simulink model "Simulation_simulink"  (R2024a)
settings: Solver=VariableStepAuto  StartTime=0.0  StopTime=reference.tsim  RelTol=1e-3
values from neighbouring files (symbols this model uses):
  Alat = Inlat_inv*Alat_    [create_sf_lti.m]
  Alon = Inlon_inv*Alon_    [create_sf_lti.m]
  Blat = Inlat_inv*Blat_    [create_sf_lti.m]
  Blon = Inlon_inv*Blon_    [create_sf_lti.m]
  Kd_psi = 10    [Mh03_h1000.m]    (also in demo.m)
  Kd_roll = -10    [Mh03_h1000.m]    (also in demo.m)
  Ki_pitch = -0.1    [Mh03_h1000.m]    (also in demo.m)
  Ki_psi = 0.1    [Mh03_h1000.m]    (also in demo.m)
  Kp = -4.7989    [Mh03_h1000.m]    (also in controller_1.m = evalin("base", "Kp"); demo.m)
  Kp_pitch = -10    [Mh03_h1000.m]    (also in demo.m = -1)
  Kp_psi = 10    [Mh03_h1000.m]    (also in demo.m)
  Kp_roll = -1    [Mh03_h1000.m]    (also in demo.m)
  Kq = -100000    [Mh03_h1000.m]    (also in controller_1.m = evalin("base", "Kq"); demo.m = 100)
  Kr = 6.9343    [Mh03_h1000.m]    (also in controller_1.m = evalin("base", "Kr"); demo.m)
  Ksp = 0.1    [Mh03_h1000.m]    (also in demo.m)
  Ksq = 0.1    [Mh03_h1000.m]    (also in demo.m)
  Ksr = 0.1    [Mh03_h1000.m]    (also in demo.m)
  reference = evalin('base', 'reference')    [GravityFM.m]    (also in Mh03_h1000.m = create_sf_reference(); demo.m = create_sf_reference())
  tau_p = 0.5    [Mh03_h1000.m]    (also in demo.m)
  tau_q = 0.5    [Mh03_h1000.m]    (also in demo.m)
  tau_r = 0.5    [Mh03_h1000.m]    (also in demo.m)
undefined symbols (not defined in the file or in its folder): Earth, Kiq, Kpp, Kpq, Kpr, KSp, KSr, WGS84
libraries: slpidlib x2, aerolibtransform2 x1
settings Model: Creator=jelho  LastModifiedBy=ludhor
settings DataIOCC: ExternalInput=getinputstruct(report2)  InitialState=getstatestruct(report2)
settings RTWCC: GPUComputeCapability=3.5

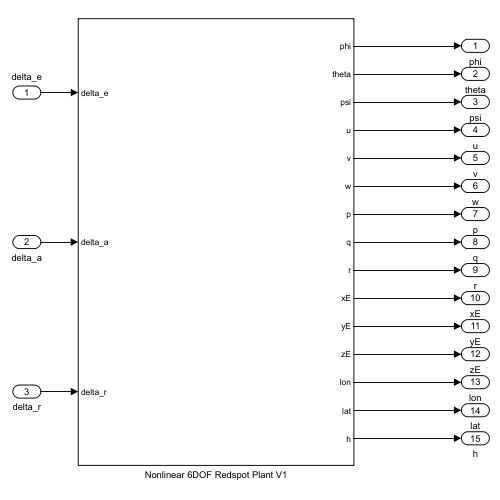
[thumbnail: Simulink's stored preview of the top-level diagram]
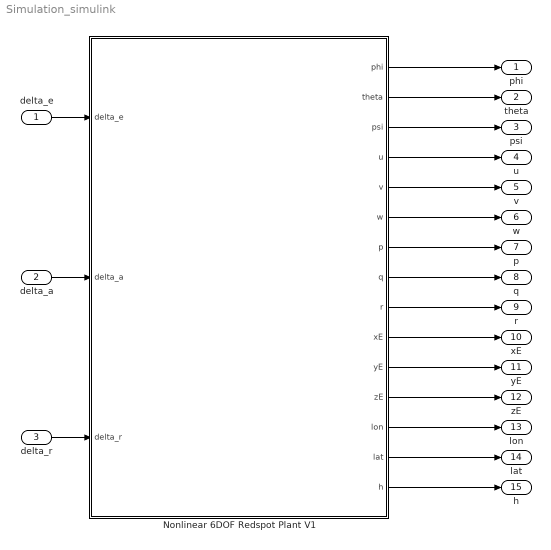
== system Simulation_simulink ==
  delta_e : Inport
  delta_a : Inport  Port=2
  delta_r : Inport  Port=3
  Nonlinear 6DOF Redspot Plant V1 : Subsystem
  phi : Outport
  theta : Outport  Port=2
  psi : Outport  Port=3
  u : Outport  Port=4
  v : Outport  Port=5
  w : Outport  Port=6
  p : Outport  Port=7
  q : Outport  Port=8
  r : Outport  Port=9
  xE : Outport  Port=10
  yE : Outport  Port=11
  zE : Outport  Port=12
  lon : Outport  Port=13
  lat : Outport  Port=14
  h : Outport  Port=15
  wires:
  delta_e/1 -> Nonlinear 6DOF Redspot Plant V1/1(delta_e)
  delta_a/1 -> Nonlinear 6DOF Redspot Plant V1/2(delta_a)
  delta_r/1 -> Nonlinear 6DOF Redspot Plant V1/3(delta_r)
  Nonlinear 6DOF Redspot Plant V1/6(w) -> w/1
  Nonlinear 6DOF Redspot Plant V1/1(phi) -> phi/1
  Nonlinear 6DOF Redspot Plant V1/4(u) -> u/1
  Nonlinear 6DOF Redspot Plant V1/2(theta) -> theta/1
  Nonlinear 6DOF Redspot Plant V1/3(psi) -> psi/1
  Nonlinear 6DOF Redspot Plant V1/5(v) -> v/1
  Nonlinear 6DOF Redspot Plant V1/7(p) -> p/1
  Nonlinear 6DOF Redspot Plant V1/8(q) -> q/1
  Nonlinear 6DOF Redspot Plant V1/9(r) -> r/1
  Nonlinear 6DOF Redspot Plant V1/10(xE) -> xE/1
  Nonlinear 6DOF Redspot Plant V1/11(yE) -> yE/1
  Nonlinear 6DOF Redspot Plant V1/12(zE) -> zE/1
  Nonlinear 6DOF Redspot Plant V1/13(lon) -> lon/1
  Nonlinear 6DOF Redspot Plant V1/14(lat) -> lat/1
  Nonlinear 6DOF Redspot Plant V1/15(h) -> h/1

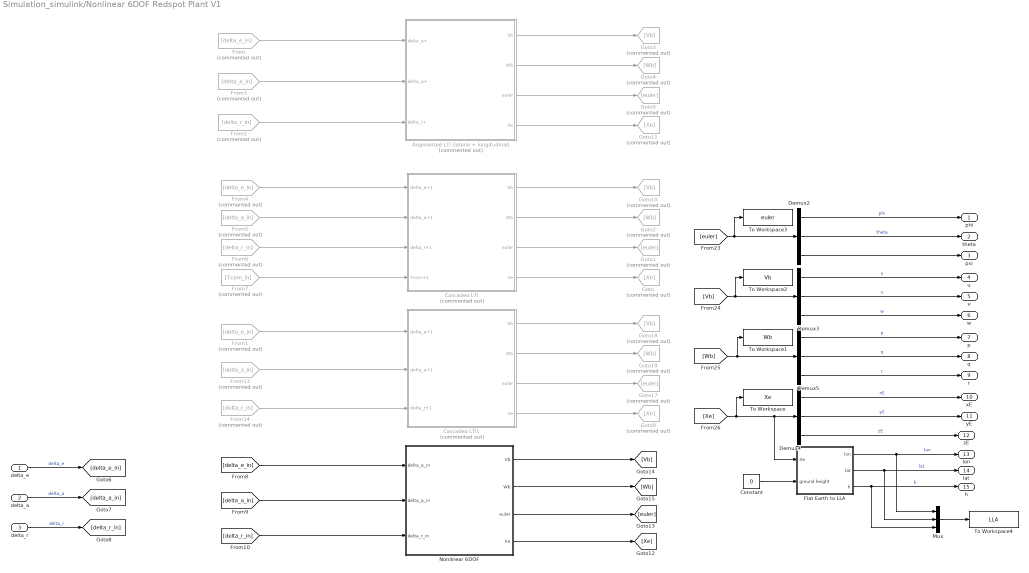
== system Simulation_simulink/Nonlinear 6DOF Redspot Plant V1 ==
  delta_e : Inport
  delta_a : Inport  Port=2
  delta_r : Inport  Port=3
  Augmented LTI (lateral + longitudinal) : Subsystem  Commented=on
  Cascaded LTI : Subsystem  Commented=on
  Cascaded LTI1 : Subsystem  Commented=on
  Constant : Constant  Value=0
  Demux{2..5} (4 alike) : Demux  Outputs=3
  Flat Earth to LLA : Subsystem
  From : From  Commented=on  GotoTag=delta_e_in
  From1 : From  Commented=on  GotoTag=delta_e_in
  From13 : From  Commented=on  GotoTag=delta_a_in
  From14 : From  Commented=on  GotoTag=delta_r_in
  From2 : From  Commented=on  GotoTag=delta_r_in
  From3 : From  Commented=on  GotoTag=delta_a_in
  From4 : From  Commented=on  GotoTag=delta_e_in
  From5 : From  Commented=on  GotoTag=delta_a_in
  From6 : From  Commented=on  GotoTag=delta_r_in
  From7 : From  Commented=on  GotoTag=Tcom_in
  Goto : Goto  Commented=on  GotoTag=Xe
  Goto1 : Goto  Commented=on  GotoTag=euler
  Goto10 : Goto  Commented=on  GotoTag=Vb
  Goto11 : Goto  Commented=on  GotoTag=Xe
  Goto17 : Goto  Commented=on  GotoTag=euler
  Goto18 : Goto  Commented=on  GotoTag=Vb
  Goto19 : Goto  Commented=on  GotoTag=Wb
  Goto2 : Goto  Commented=on  GotoTag=Wb
  Goto3 : Goto  Commented=on  GotoTag=Vb
  Goto4 : Goto  Commented=on  GotoTag=Wb
  Goto5 : Goto  Commented=on  GotoTag=euler
  Goto9 : Goto  Commented=on  GotoTag=Xe
  Mux : Mux  Inputs=3
  Nonlinear 6DOF : Subsystem
  To Workspace : ToWorkspace  VariableName=Xe  SaveFormat=Timeseries  SampleTime=-1
  To Workspace1 : ToWorkspace  VariableName=Wb  SaveFormat=Timeseries  SampleTime=-1
  To Workspace2 : ToWorkspace  VariableName=Vb  SaveFormat=Timeseries  SampleTime=-1
  To Workspace3 : ToWorkspace  VariableName=euler  SaveFormat=Timeseries  SampleTime=-1
  To Workspace4 : ToWorkspace  VariableName=LLA  SaveFormat=Timeseries  SampleTime=-1
  phi : Outport
  theta : Outport  Port=2
  psi : Outport  Port=3
  u : Outport  Port=4
  v : Outport  Port=5
  w : Outport  Port=6
  p : Outport  Port=7
  q : Outport  Port=8
  r : Outport  Port=9
  xE : Outport  Port=10
  yE : Outport  Port=11
  zE : Outport  Port=12
  lon : Outport  Port=13
  lat : Outport  Port=14
  h : Outport  Port=15
  wires:
  delta_a/1 -> [delta_a_in]  "delta_a"
  delta_e/1 -> [delta_e_in]  "delta_e"
  [Vb] -> To Workspace2/1, Demux3/1
  [euler] -> To Workspace3/1, Demux2/1
  delta_r/1 -> [delta_r_in]  "delta_r"
  Demux2/1 -> phi/1  "phi"
  Demux2/2 -> theta/1  "theta"
  Demux2/3 -> psi/1
  Demux3/3 -> w/1  "w"
  Demux3/1 -> u/1  "u"
  Demux3/2 -> v/1  "v"
  Demux5/2 -> q/1  "q"
  [Wb] -> To Workspace1/1, Demux5/1
  Demux5/1 -> p/1  "p"
  Demux5/3 -> r/1  "r"
  [Xe] -> To Workspace/1, Flat Earth to LLA/1(Xe), Demux4/1
  Demux4/2 -> yE/1  "yE"
  Demux4/3 -> zE/1  "zE"
  Demux4/1 -> xE/1  "xE"
  [delta_e_in] -> Nonlinear 6DOF/1(delta_e_in)
  [delta_a_in] -> Nonlinear 6DOF/2(delta_a_in)
  [delta_r_in] -> Nonlinear 6DOF/3(delta_r_in)
  Nonlinear 6DOF/1(Vb) -> [Vb]
  Nonlinear 6DOF/2(Wb) -> [Wb]
  Nonlinear 6DOF/3(euler) -> [euler]
  Nonlinear 6DOF/4(Xe) -> [Xe]
  From4/1 -> Cascaded LTI/1(delta_e+1)
  From5/1 -> Cascaded LTI/2(delta_a+1)
  From6/1 -> Cascaded LTI/3(delta_r+1)
  From7/1 -> Cascaded LTI/4(Tcom+1)
  Cascaded LTI/1(Vb) -> Goto10/1
  Cascaded LTI/2(Wb) -> Goto2/1
  Cascaded LTI/3(euler) -> Goto1/1
  Cascaded LTI/4(Xe) -> Goto/1
  From/1 -> Augmented LTI (lateral + longitudinal)/1(delta_e+)
  From2/1 -> Augmented LTI (lateral + longitudinal)/3(delta_r+)
  From3/1 -> Augmented LTI (lateral + longitudinal)/2(delta_a+)
  Augmented LTI (lateral + longitudinal)/1(Vb) -> Goto3/1
  Augmented LTI (lateral + longitudinal)/2(Wb) -> Goto4/1
  Augmented LTI (lateral + longitudinal)/3(euler) -> Goto5/1
  Augmented LTI (lateral + longitudinal)/4(Xe) -> Goto11/1
  Flat Earth to LLA/1(lon) -> Mux/1, lon/1  "lon"
  Flat Earth to LLA/2(lat) -> Mux/2, lat/1  "lat"
  Flat Earth to LLA/3(h) -> Mux/3, h/1  "h"
  Constant/1 -> Flat Earth to LLA/2(ground height)
  Mux/1 -> To Workspace4/1
  From1/1 -> Cascaded LTI1/1(delta_e+1)
  Cascaded LTI1/4(Xe) -> Goto9/1
  Cascaded LTI1/1(Vb) -> Goto18/1
  From14/1 -> Cascaded LTI1/3(delta_r+1)
  From13/1 -> Cascaded LTI1/2(delta_a+1)
  Cascaded LTI1/3(euler) -> Goto17/1
  Cascaded LTI1/2(Wb) -> Goto19/1

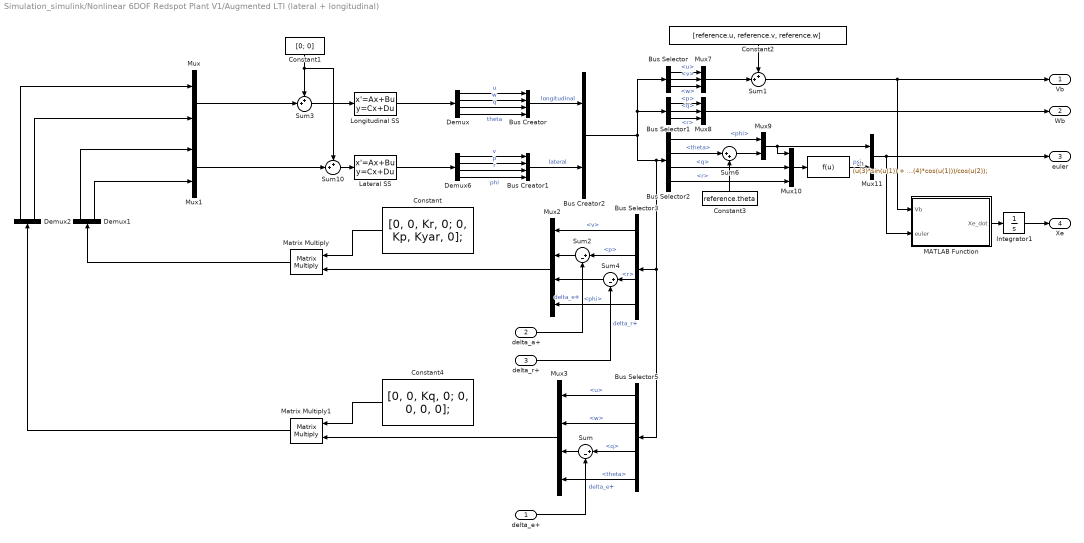
== system Simulation_simulink/Nonlinear 6DOF Redspot Plant V1/Augmented LTI (lateral + longitudinal) ==
  delta_e+ : Inport
  delta_a+ : Inport  Port=2
  delta_r+ : Inport  Port=3
  Bus Creator : BusCreator  Inputs=4
  Bus Creator1 : BusCreator  Inputs=4
  Bus Creator2 : BusCreator  Inputs=2
  Bus Selector : BusSelector  OutputSignals=longitudinal.u,lateral.v,longitudinal.w
  Bus Selector1 : BusSelector  OutputSignals=lateral.p,longitudinal.q,lateral.r
  Bus Selector2 : BusSelector  OutputSignals=lateral.phi,longitudinal.theta,longitudinal.q,lateral.r
  Bus Selector3 : BusSelector  OutputSignals=lateral.v,lateral.p,lateral.r,lateral.phi
  Bus Selector5 : BusSelector  OutputSignals=longitudinal.u,longitudinal.w,longitudinal.q,longitudinal.theta
  Constant : Constant  Value=|
      | [0,  0, Kr, 0;
      | 0, Kp, Kyar, 0];
  Constant1 : Constant  Value=[0; 0]
  Constant2 : Constant  Value=[reference.u, reference.v, reference.w]
  Constant3 : Constant  Value=reference.theta
  Constant4 : Constant  Value="[0, 0, Kq, 0; 0, 0,  0, 0];"
  Demux : Demux
  Demux1 : Demux  Outputs=2
  Demux2 : Demux  Outputs=2
  Demux6 : Demux
  Fcn : Fcn  Expr=(u(3)*sin(u(1)) + u(4)*cos(u(1)))/cos(u(2));
  Integrator1 : Integrator  InitialCondition=reference.ip
  Lateral SS : StateSpace  A=Alat  B=Blat  C=eye(4)  D=zeros(4,2)  InitialCondition=0  ContinuousStateAttributes={'v', 'p', 'r', 'phi'}
  Longitudinal SS : StateSpace  A=Alon  B=Blon  C=eye(4)  D=zeros(4,2)  InitialCondition=0  ContinuousStateAttributes={'u', 'w', 'q', 'theta'}
  MATLAB Function : MATLAB Function  TreatAsAtomicUnit=on
  Matrix Multiply : Product  Multiplication=Matrix(*)
  Matrix Multiply1 : Product  Multiplication=Matrix(*)
  Mux{,1,9,11} (4 alike) : Mux  Inputs=2
  Mux10 : Mux  Inputs=3
  Mux2 : Mux
  Mux3 : Mux
  Mux7 : Mux  Inputs=3
  Mux8 : Mux  Inputs=3
  Sum : Sum  Inputs=|+-
  Sum1 : Sum  Inputs=++|
  Sum10 : Sum  Inputs=++|
  Sum2 : Sum  Inputs=|+-
  Sum3 : Sum  Inputs=++|
  Sum4 : Sum  Inputs=|+-
  Sum6 : Sum  Inputs=|++
  Vb : Outport
  Wb : Outport  Port=2
  euler : Outport  Port=3
  Xe : Outport  Port=4
  wires:
  Demux6/1 -> Bus Creator1/1  "v"
  Bus Creator2/1 -> Bus Selector5/1, Bus Selector3/1, Bus Selector2/1, Bus Selector1/1, Bus Selector/1
  Mux11/1 -> euler/1, MATLAB Function/2(euler)
  MATLAB Function/1(Xe_dot) -> Integrator1/1
  Mux9/1 -> Mux11/1, Mux10/1
  Mux10/1 -> Fcn/1
  Bus Selector1/1 -> Mux8/1  "<p>"
  Demux/1 -> Bus Creator/1  "u"
  Sum1/1 -> Vb/1, MATLAB Function/1(Vb)
  Constant3/1 -> Sum6/2
  Bus Creator1/1 -> Bus Creator2/2  "lateral"
  Demux6/2 -> Bus Creator1/2  "p"
  Mux7/1 -> Sum1/2
  Demux6/3 -> Bus Creator1/3  "r"
  Mux8/1 -> Wb/1
  Integrator1/1 -> Xe/1
  Fcn/1 -> Mux11/2  "psi"
  Bus Selector2/3 -> Mux10/2  "<q>"
  Demux6/4 -> Bus Creator1/4  "phi"
  Longitudinal SS/1 -> Demux/1
  Constant2/1 -> Sum1/1
  Demux/2 -> Bus Creator/2  "w"
  Demux/4 -> Bus Creator/4  "theta"
  Bus Creator/1 -> Bus Creator2/1  "longitudinal"
  Demux/3 -> Bus Creator/3  "q"
  Bus Selector/1 -> Mux7/1  "<u>"
  Bus Selector/2 -> Mux7/2  "<v>"
  Bus Selector/3 -> Mux7/3  "<w>"
  Bus Selector1/2 -> Mux8/2  "<q>"
  Lateral SS/1 -> Demux6/1
  Bus Selector2/4 -> Mux10/3  "<r>"
  Bus Selector2/2 -> Sum6/1  "<theta>"
  Bus Selector2/1 -> Mux9/1  "<phi>"
  Bus Selector1/3 -> Mux8/3  "<r>"
  Sum6/1 -> Mux9/2
  Sum3/1 -> Longitudinal SS/1
  Constant1/1 -> Sum10/1, Sum3/1
  Sum10/1 -> Lateral SS/1
  Mux/1 -> Sum3/2
  Mux1/1 -> Sum10/2
  Demux2/2 -> Mux/2
  Demux1/1 -> Mux1/1
  Demux1/2 -> Mux1/2
  Constant/1 -> Matrix Multiply/1
  Mux2/1 -> Matrix Multiply/2
  Bus Selector3/2 -> Sum2/1  "<p>"
  Bus Selector3/1 -> Mux2/1  "<v>"
  Bus Selector3/3 -> Sum4/1  "<r>"
  Bus Selector3/4 -> Mux2/4  "<phi>"
  Matrix Multiply/1 -> Demux1/1
  Bus Selector5/2 -> Mux3/2  "<w>"
  Mux3/1 -> Matrix Multiply1/2
  Bus Selector5/3 -> Sum/1  "<q>"
  Bus Selector5/4 -> Mux3/4  "<theta>"
  Bus Selector5/1 -> Mux3/1  "<u>"
  Constant4/1 -> Matrix Multiply1/1
  Matrix Multiply1/1 -> Demux2/1
  delta_e+/1 -> Sum/2  "delta_e+"
  Demux2/1 -> Mux/1
  Sum/1 -> Mux3/3
  Sum2/1 -> Mux2/2
  delta_a+/1 -> Sum2/2  "delta_e+"
  Sum4/1 -> Mux2/3
  delta_r+/1 -> Sum4/2  "delta_r+"

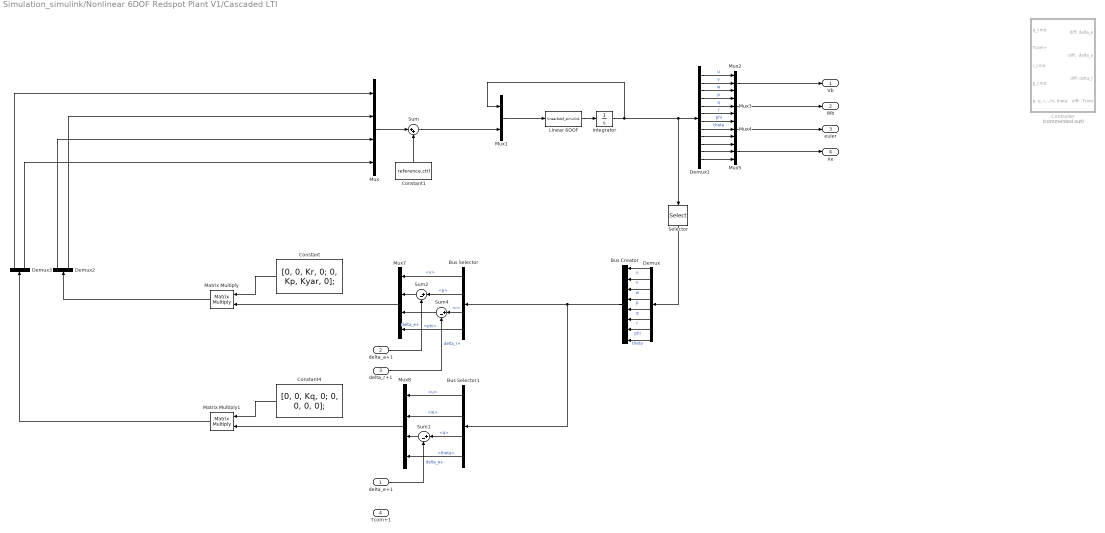
== system Simulation_simulink/Nonlinear 6DOF Redspot Plant V1/Cascaded LTI ==
  delta_e+1 : Inport
  delta_a+1 : Inport  Port=2
  delta_r+1 : Inport  Port=3
  Tcom+1 : Inport  Port=4
  Bus Creator : BusCreator  Inputs=8
  Bus Selector : BusSelector  OutputSignals=v,p,r,phi
  Bus Selector1 : BusSelector  OutputSignals=u,w,q,theta
  Constant : Constant  Value=|
      | [0,  0, Kr, 0;
      | 0, Kp, Kyar, 0];
  Constant1 : Constant  Value=reference.ctrl
  Constant4 : Constant  Value="[0, 0, Kq, 0; 0, 0,  0, 0];"
  Controller : Subsystem  Commented=on
  Demux : Demux  Outputs=8
  Demux1 : Demux  Outputs=12
  Demux2 : Demux  Outputs=2
  Demux3 : Demux  Outputs=2
  Integrator : Integrator  InitialCondition=reference.x  ContinuousStateAttributes={'u', 'v', 'w', 'p', 'q', 'r', 'phi', 'theta', 'psi', 'xE', 'yE', 'zE'}
  Linear 6DOF : MATLABFcn  MATLABFcn=linear6dof_simulink
  Matrix Multiply : Product  Multiplication=Matrix(*)
  Matrix Multiply1 : Product  Multiplication=Matrix(*)
  Mux : Mux
  Mux1 : Mux  Inputs=2
  Mux{2..5} (4 alike) : Mux  Inputs=3
  Mux7 : Mux
  Mux8 : Mux
  Selector : Selector  InputPortWidth=12  IndexOptions=Index vector (dialog)  Indices=[1 2 3 4 5 6 7 8]  OutputSizes=1
  Sum : Sum  Inputs=|++
  Sum1 : Sum  Inputs=|+-
  Sum2 : Sum  Inputs=|+-
  Sum4 : Sum  Inputs=|+-
  Vb : Outport
  Wb : Outport  Port=2
  euler : Outport  Port=3
  Xe : Outport  Port=4
  wires:
  Demux1/9 -> Mux4/3
  Mux4/1 -> euler/1
  Demux1/3 -> Mux2/3  "w"
  Demux1/12 -> Mux5/3
  Demux1/5 -> Mux3/2  "q"
  Demux1/8 -> Mux4/2  "theta"
  Mux/1 -> Sum/1
  Demux1/1 -> Mux2/1  "u"
  Demux1/11 -> Mux5/2
  Demux1/10 -> Mux5/1
  Demux1/2 -> Mux2/2  "v"
  Linear 6DOF/1 -> Integrator/1
  Demux1/4 -> Mux3/1  "p"
  Demux1/6 -> Mux3/3  "r"
  Integrator/1 -> Demux1/1, Selector/1, Mux1/1
  Constant1/1 -> Sum/2
  Demux1/7 -> Mux4/1  "phi"
  Mux3/1 -> Wb/1
  Sum/1 -> Mux1/2
  Mux1/1 -> Linear 6DOF/1
  Mux2/1 -> Vb/1
  Mux5/1 -> Xe/1
  Demux3/1 -> Mux/1
  Demux2/1 -> Mux/3
  Demux3/2 -> Mux/4
  Mux7/1 -> Matrix Multiply/2
  delta_e+1/1 -> Sum1/2  "delta_e+"
  Sum2/1 -> Mux7/2
  delta_r+1/1 -> Sum4/2  "delta_r+"
  delta_a+1/1 -> Sum2/2  "delta_e+"
  Constant4/1 -> Matrix Multiply1/1
  Matrix Multiply/1 -> Demux2/1
  Bus Selector/4 -> Mux7/4  "<phi>"
  Demux2/2 -> Mux/2
  Bus Selector/1 -> Mux7/1  "<v>"
  Bus Selector1/4 -> Mux8/4  "<theta>"
  Bus Selector1/2 -> Mux8/2  "<w>"
  Mux8/1 -> Matrix Multiply1/2
  Matrix Multiply1/1 -> Demux3/1
  Sum1/1 -> Mux8/3
  Bus Selector1/3 -> Sum1/1  "<q>"
  Sum4/1 -> Mux7/3
  Bus Selector/2 -> Sum2/1  "<p>"
  Constant/1 -> Matrix Multiply/1
  Bus Selector/3 -> Sum4/1  "<r>"
  Bus Selector1/1 -> Mux8/1  "<u>"
  Demux/1 -> Bus Creator/1  "u"
  Demux/2 -> Bus Creator/2  "v"
  Demux/3 -> Bus Creator/3  "w"
  Demux/4 -> Bus Creator/4  "p"
  Demux/5 -> Bus Creator/5  "q"
  Demux/6 -> Bus Creator/6  "r"
  Demux/7 -> Bus Creator/7  "phi"
  Demux/8 -> Bus Creator/8  "theta"
  Bus Creator/1 -> Bus Selector1/1, Bus Selector/1
  Selector/1 -> Demux/1

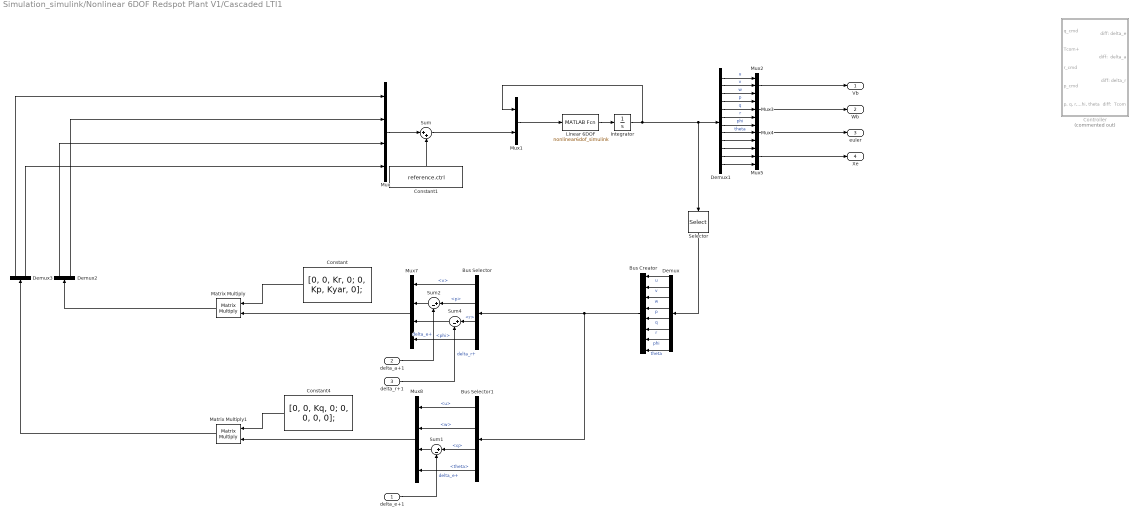
== system Simulation_simulink/Nonlinear 6DOF Redspot Plant V1/Cascaded LTI1 ==
  delta_e+1 : Inport
  delta_a+1 : Inport  Port=2
  delta_r+1 : Inport  Port=3
  Bus Creator : BusCreator  Inputs=8
  Bus Selector : BusSelector  OutputSignals=v,p,r,phi
  Bus Selector1 : BusSelector  OutputSignals=u,w,q,theta
  Constant : Constant  Value=|
      | [0,  0, Kr, 0;
      | 0, Kp, Kyar, 0];
  Constant1 : Constant  Value=reference.ctrl
  Constant4 : Constant  Value="[0, 0, Kq, 0; 0, 0,  0, 0];"
  Controller : Subsystem  Commented=on
  Demux : Demux  Outputs=8
  Demux1 : Demux  Outputs=12
  Demux2 : Demux  Outputs=2
  Demux3 : Demux  Outputs=2
  Integrator : Integrator  InitialCondition=reference.x  ContinuousStateAttributes={'u', 'v', 'w', 'p', 'q', 'r', 'phi', 'theta', 'psi', 'xE', 'yE', 'zE'}
  Linear 6DOF : MATLABFcn  MATLABFcn=nonlinear6dof_simulink
  Matrix Multiply : Product  Multiplication=Matrix(*)
  Matrix Multiply1 : Product  Multiplication=Matrix(*)
  Mux : Mux
  Mux1 : Mux  Inputs=2
  Mux{2..5} (4 alike) : Mux  Inputs=3
  Mux7 : Mux
  Mux8 : Mux
  Selector : Selector  InputPortWidth=12  IndexOptions=Index vector (dialog)  Indices=[1 2 3 4 5 6 7 8]  OutputSizes=1
  Sum : Sum  Inputs=|++
  Sum1 : Sum  Inputs=|+-
  Sum2 : Sum  Inputs=|+-
  Sum4 : Sum  Inputs=|+-
  Vb : Outport
  Wb : Outport  Port=2
  euler : Outport  Port=3
  Xe : Outport  Port=4
  wires:
  Demux1/9 -> Mux4/3
  Mux4/1 -> euler/1
  Demux1/3 -> Mux2/3  "w"
  Demux1/12 -> Mux5/3
  Demux1/5 -> Mux3/2  "q"
  Demux1/8 -> Mux4/2  "theta"
  Mux/1 -> Sum/1
  Demux1/1 -> Mux2/1  "u"
  Demux1/11 -> Mux5/2
  Demux1/10 -> Mux5/1
  Demux1/2 -> Mux2/2  "v"
  Linear 6DOF/1 -> Integrator/1
  Demux1/4 -> Mux3/1  "p"
  Demux1/6 -> Mux3/3  "r"
  Integrator/1 -> Demux1/1, Selector/1, Mux1/1
  Constant1/1 -> Sum/2
  Demux1/7 -> Mux4/1  "phi"
  Mux3/1 -> Wb/1
  Sum/1 -> Mux1/2
  Mux1/1 -> Linear 6DOF/1
  Mux2/1 -> Vb/1
  Mux5/1 -> Xe/1
  Demux3/1 -> Mux/1
  Demux2/1 -> Mux/3
  Demux3/2 -> Mux/4
  Mux7/1 -> Matrix Multiply/2
  delta_e+1/1 -> Sum1/2  "delta_e+"
  Sum2/1 -> Mux7/2
  delta_r+1/1 -> Sum4/2  "delta_r+"
  delta_a+1/1 -> Sum2/2  "delta_e+"
  Constant4/1 -> Matrix Multiply1/1
  Matrix Multiply/1 -> Demux2/1
  Bus Selector/4 -> Mux7/4  "<phi>"
  Demux2/2 -> Mux/2
  Bus Selector/1 -> Mux7/1  "<v>"
  Bus Selector1/4 -> Mux8/4  "<theta>"
  Bus Selector1/2 -> Mux8/2  "<w>"
  Mux8/1 -> Matrix Multiply1/2
  Matrix Multiply1/1 -> Demux3/1
  Sum1/1 -> Mux8/3
  Bus Selector1/3 -> Sum1/1  "<q>"
  Sum4/1 -> Mux7/3
  Bus Selector/2 -> Sum2/1  "<p>"
  Bus Selector/3 -> Sum4/1  "<r>"
  Bus Selector1/1 -> Mux8/1  "<u>"
  Demux/1 -> Bus Creator/1  "u"
  Demux/2 -> Bus Creator/2  "v"
  Demux/3 -> Bus Creator/3  "w"
  Demux/4 -> Bus Creator/4  "p"
  Demux/5 -> Bus Creator/5  "q"
  Demux/6 -> Bus Creator/6  "r"
  Demux/7 -> Bus Creator/7  "phi"
  Demux/8 -> Bus Creator/8  "theta"
  Bus Creator/1 -> Bus Selector1/1, Bus Selector/1
  Selector/1 -> Demux/1
  Constant/1 -> Matrix Multiply/1

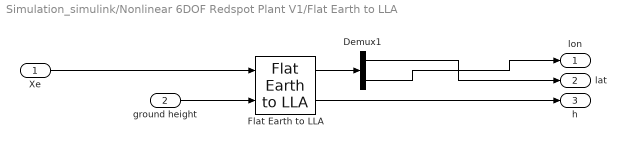
== system Simulation_simulink/Nonlinear 6DOF Redspot Plant V1/Flat Earth to LLA ==
  Xe : Inport
  ground height : Inport  Port=2
  Demux1 : Demux  Outputs=2
  Flat Earth to LLA : aerolibtransform2/Flat Earth to LLA  units=Metric (MKS)  ptype=Earth (WGS84)  F=1/298.257223563  R=6378137  refPosPort=off  LL0=[reference.latitude reference.longitude]  psi=0
  lon : Outport
  lat : Outport  Port=2
  h : Outport  Port=3
  wires:
  Flat Earth to LLA/2 -> h/1
  ground height/1 -> Flat Earth to LLA/2
  Flat Earth to LLA/1 -> Demux1/1
  Demux1/2 -> lon/1
  Xe/1 -> Flat Earth to LLA/1
  Demux1/1 -> lat/1

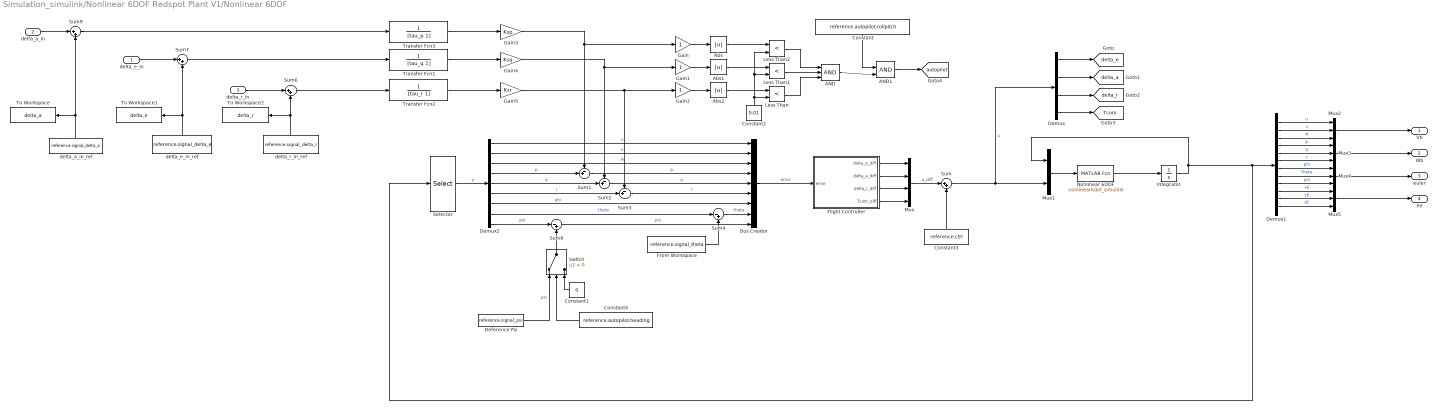
== system Simulation_simulink/Nonlinear 6DOF Redspot Plant V1/Nonlinear 6DOF ==
  delta_e_in : Inport
  delta_a_in : Inport  Port=2
  delta_r_in : Inport  Port=3
  AND : Logic  Inputs=3  IconShape=distinctive  AllPortsSameDT=off  OutDataTypeStr=boolean
  AND1 : Logic  IconShape=distinctive  AllPortsSameDT=off  OutDataTypeStr=boolean
  Abs : Abs  SaturateOnIntegerOverflow=off
  Abs1 : Abs  SaturateOnIntegerOverflow=off
  Abs2 : Abs  SaturateOnIntegerOverflow=off
  Bus Creator : BusCreator  Inputs=9
  Constant : Constant  Value=reference.autopilot.rollpitch
  Constant1 : Constant  Value=0
  Constant2 : Constant  Value=0.01
  Constant3 : Constant  Value=reference.ctrl
  Constant4 : Constant  Value=reference.autopilot.heading
  Demux : Demux
  Demux1 : Demux  Outputs=12
  Demux2 : Demux  Outputs=9
  Flight Controller : Subsystem
  From Workspace : FromWorkspace  VariableName=reference.signal_theta
  Gain : Gain
  Gain1 : Gain
  Gain2 : Gain
  Gain3 : Gain  Gain=Ksp
  Gain4 : Gain  Gain=Ksq
  Gain5 : Gain  Gain=Ksr
  Integrator : Integrator  InitialCondition=reference.x  ContinuousStateAttributes={'u', 'v', 'w', 'p', 'q', 'r', 'phi', 'theta', 'psi', 'xE', 'yE', 'zE'}
  Less Than : RelationalOperator  Operator=<  OutDataTypeStr=boolean  RndMeth=Simplest  InputSameDT=off
  Less Than1 : RelationalOperator  Operator=<  OutDataTypeStr=boolean  RndMeth=Simplest  InputSameDT=off
  Less Than2 : RelationalOperator  Operator=<  OutDataTypeStr=boolean  RndMeth=Simplest  InputSameDT=off
  Mux : Mux
  Mux1 : Mux  Inputs=2
  Mux{2..5} (4 alike) : Mux  Inputs=3
  Nonlinear 6DOF : MATLABFcn  MATLABFcn=nonlinear6dof_simulink
  Reference Psi : FromWorkspace  VariableName=reference.signal_psi
  Selector : Selector  InputPortWidth=12  IndexOptions=Index vector (dialog)  Indices=[1 2 3 4 5 6 7 8 9]  OutputSizes=1
  Sum{,6..7,9} (4 alike) : Sum  Inputs=|++
  Sum1 : Sum  Inputs=-+|
  Sum2 : Sum  Inputs=-+|
  Sum3 : Sum  Inputs=-+|
  Sum4 : Sum  Inputs=|-+
  Sum8 : Sum  Inputs=|-+
  Switch : Switch  Criteria=u2 > Threshold  SaturateOnIntegerOverflow=off  InputSameDT=off
  To Workspace : ToWorkspace  VariableName=delta_a  SaveFormat=Timeseries  SampleTime=-1
  To Workspace1 : ToWorkspace  VariableName=delta_e  SaveFormat=Timeseries  SampleTime=-1
  To Workspace2 : ToWorkspace  VariableName=delta_r  SaveFormat=Timeseries  SampleTime=-1
  Transfer Fcn1 : TransferFcn  Denominator=[tau_q 1]
  Transfer Fcn2 : TransferFcn  Denominator=[tau_r 1]
  Transfer Fcn3 : TransferFcn  Denominator=[tau_p 1]
  delta_a_in_ref : FromWorkspace  VariableName=reference.signal_delta_a  OutputAfterFinalValue=Holding final value
  delta_e_in_ref : FromWorkspace  VariableName=reference.signal_delta_e  OutputAfterFinalValue=Holding final value
  delta_r_in_ref : FromWorkspace  VariableName=reference.signal_delta_r  OutputAfterFinalValue=Holding final value
  Vb : Outport
  Wb : Outport  Port=2
  euler : Outport  Port=3
  Xe : Outport  Port=4
  tag scope: Tcom=global, autopilot=global, delta_a=global, delta_e=global, delta_r=global
  wires:
  Mux5/1 -> Xe/1
  Nonlinear 6DOF/1 -> Integrator/1
  Constant3/1 -> Sum/2
  Mux2/1 -> Vb/1
  Mux1/1 -> Nonlinear 6DOF/1
  Demux1/12 -> Mux5/3  "zE"
  Demux1/7 -> Mux4/1  "phi"
  Demux1/2 -> Mux2/2  "v"
  Demux1/6 -> Mux3/3  "r"
  Mux3/1 -> Wb/1
  Demux1/4 -> Mux3/1  "p"
  Demux1/10 -> Mux5/1  "xE"
  Demux1/11 -> Mux5/2  "yE"
  Mux/1 -> Sum/1  "u_diff"
  Demux1/9 -> Mux4/3  "psi"
  Demux1/3 -> Mux2/3  "w"
  Demux1/8 -> Mux4/2  "theta"
  Mux4/1 -> euler/1
  Demux1/1 -> Mux2/1  "u"
  Demux1/5 -> Mux3/2  "q"
  Demux/3 -> [delta_r]
  Demux/1 -> [delta_e]
  Demux/2 -> [delta_a]
  Demux/4 -> [Tcom]
  Sum/1 -> Demux/1, Mux1/2  "u"
  Selector/1 -> Demux2/1  "y"
  Demux2/7 -> Bus Creator/7  "phi"
  Demux2/6 -> Sum3/2  "r"
  Demux2/4 -> Sum1/2  "p"
  Demux2/1 -> Bus Creator/1  "u"
  Demux2/3 -> Bus Creator/3  "w"
  Demux2/2 -> Bus Creator/2  "v"
  Demux2/5 -> Sum2/2  "q"
  Demux2/8 -> Sum4/1  "theta"
  Flight Controller/1(delta_e_diff) -> Mux/1
  Flight Controller/2(delta_a_diff) -> Mux/2
  Flight Controller/3(delta_r_diff) -> Mux/3
  Flight Controller/4(Tcom_diff) -> Mux/4
  Bus Creator/1 -> Flight Controller/1(error)  "error"
  Sum1/1 -> Bus Creator/4  "p"
  Sum2/1 -> Bus Creator/5  "q"
  Sum3/1 -> Bus Creator/6  "r"
  Sum4/1 -> Bus Creator/8  "theta"
  Gain/1 -> Abs/1
  Gain1/1 -> Abs1/1
  Gain2/1 -> Abs2/1
  Abs/1 -> Less Than2/1
  Constant2/1 -> Less Than/2, Less Than2/2, Less Than1/2
  Abs1/1 -> Less Than1/1
  Less Than/1 -> AND/3
  Abs2/1 -> Less Than/1
  Less Than2/1 -> AND/1
  Less Than1/1 -> AND/2
  AND/1 -> AND1/2
  AND1/1 -> [autopilot]
  Constant/1 -> AND1/1
  Transfer Fcn3/1 -> Gain3/1
  Transfer Fcn1/1 -> Gain4/1
  Transfer Fcn2/1 -> Gain5/1
  Gain3/1 -> Sum1/1, Gain/1
  Gain4/1 -> Gain1/1, Sum2/1
  Gain5/1 -> Gain2/1, Sum3/1
  From Workspace/1 -> Sum4/2
  delta_r_in/1 -> Sum6/1
  delta_e_in/1 -> Sum7/1
  delta_a_in/1 -> Sum9/1
  Demux2/9 -> Sum8/1  "psi"
  Sum8/1 -> Bus Creator/9  "psi"
  Integrator/1 -> Demux1/1, Selector/1, Mux1/1
  Reference Psi/1 -> Switch/1  "psi"
  Sum6/1 -> Transfer Fcn2/1
  delta_r_in_ref/1 -> To Workspace2/1, Sum6/2
  Sum7/1 -> Transfer Fcn1/1
  delta_e_in_ref/1 -> Sum7/2, To Workspace1/1
  delta_a_in_ref/1 -> Sum9/2, To Workspace/1
  Sum9/1 -> Transfer Fcn3/1
  Constant1/1 -> Switch/3
  Constant4/1 -> Switch/2
  Switch/1 -> Sum8/2

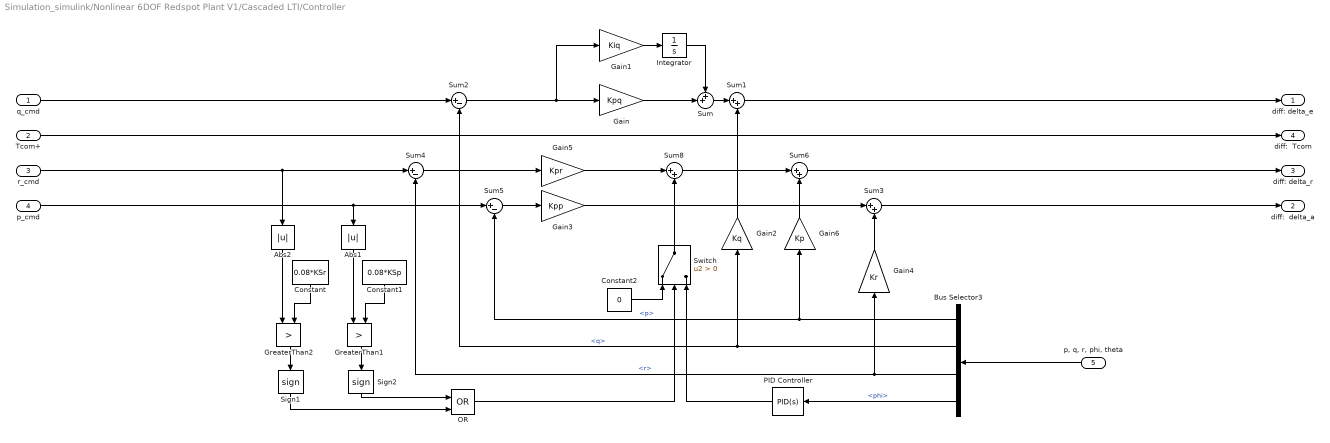
== system Simulation_simulink/Nonlinear 6DOF Redspot Plant V1/Cascaded LTI/Controller ==
  q_cmd : Inport
  Tcom+ : Inport  Port=2
  r_cmd : Inport  Port=3
  p_cmd : Inport  Port=4
  "p, q, r, phi, theta" : Inport  Port=5
  Abs1 : Abs  SaturateOnIntegerOverflow=off
  Abs2 : Abs  SaturateOnIntegerOverflow=off
  Bus Selector3 : BusSelector  OutputSignals=p,q,r,phi
  Constant : Constant  Value=0.08*KSr
  Constant1 : Constant  Value=0.08*KSp
  Constant2 : Constant  Value=0
  Gain : Gain  Gain=Kpq
  Gain1 : Gain  Gain=Kiq
  Gain2 : Gain  Gain=Kq
  Gain3 : Gain  Gain=Kpp
  Gain4 : Gain  Gain=Kr
  Gain5 : Gain  Gain=Kpr
  Gain6 : Gain  Gain=Kp
  GreaterThan1 : RelationalOperator  Operator=>  OutDataTypeStr=boolean  RndMeth=Simplest  InputSameDT=off
  GreaterThan2 : RelationalOperator  Operator=>  OutDataTypeStr=boolean  RndMeth=Simplest  InputSameDT=off
  Integrator : Integrator
  OR : Logic  Operator=OR  IconShape=distinctive  AllPortsSameDT=off  OutDataTypeStr=boolean
  PID Controller : slpidlib/PID Controller  Controller=PID  Form=Parallel  TimeDomain=Continuous-time  UseExternalTs=off  SampleTime=-1  IntegratorMethod=Forward Euler  FilterMethod=Forward Euler  ControllerParametersSource=internal  P=10  I=0.5  UseKiTs=off  D=5  N=100  UseFilter=on  TunerSelectOption=Transfer Function Based (PID Tuner App)  InitialConditionSource=internal  InitialConditionForIntegrator=0  InitialConditionForFilter=0  DifferentiatorICPrevScaledInput=0  ExternalReset=none  TrackingMode=off  Kt=1  LimitOutput=off  SatLimitsSource=internal  UpperSaturationLimit=inf  LowerSaturationLimit=-inf  LinearizeAsGain=on  AntiWindupMode=none  Kb=1  LimitIntegrator=off  UpperIntegratorSaturationLimit=inf  LowerIntegratorSaturationLimit=-inf  POutMin=[]  POutMax=[]  IOutMin=[]  IOutMax=[]  DOutMin=[]  DOutMax=[]  NOutMin=[]  NOutMax=[]  SumOutMin=[]  SumOutMax=[]  SaturationOutMin=[]  SaturationOutMax=[]  PParamMin=[]  PParamMax=[]  IParamMin=[]  IParamMax=[]  DParamMin=[]  DParamMax=[]  NParamMin=[]  NParamMax=[]  KbParamMin=[]  KbParamMax=[]  KtParamMin=[]  KtParamMax=[]  KbOutMin=[]  KbOutMax=[]  KtOutMin=[]  KtOutMax=[]  IntegratorOutMin=[]  IntegratorOutMax=[]  FilterOutMin=[]  FilterOutMax=[]  SumI1OutMin=[]  SumI1OutMax=[]  SumI2OutMin=[]  SumI2OutMax=[]  SumI3OutMin=[]  SumI3OutMax=[]  SumI4OutMin=[]  SumI4OutMax=[]  SumDOutMin=[]  SumDOutMax=[]  DifferentiatorOutMin=[]  DifferentiatorOutMax=[]  FilterDiffOutCoefMin=[]  FilterDiffOutCoefMax=[]  ReciprocalOutMin=[]  ReciprocalOutMax=[]  SumDenOutMin=[]  SumDenOutMax=[]  SumNumOutMin=[]  SumNumOutMax=[]  DivideOutMin=[]  DivideOutMax=[]  UdiffTsProdOutMin=[]  UdiffTsProdOutMax=[]  NTsProdOutMin=[]  NTsProdOutMax=[]  UintegralTsProdOutMin=[]  UintegralTsProdOutMax=[]  UngainTsProdOutMin=[]  UngainTsProdOutMax=[]  ClampingZeroOutDataTypeStr=Inherit: Inherit via back propagation  ClampingZeroOutMin=[]  ClampingZeroOutMax=[]  FilterDenConstantOutDataTypeStr=Inherit: Inherit via back propagation  FilterDenConstantOutMin=[]  FilterDenConstantOutMax=[]  PCopyOutDataTypeStr=Inherit: Inherit via back propagation  PCopyOutMin=[]  PCopyOutMax=[]  NCopyOutDataTypeStr=Inherit: Inherit via back propagation  NCopyOutMin=[]  NCopyOutMax=[]  IntegratorContinuousStateAttributes=''  IntegratorStateMustResolveToSignalObject=off  IntegratorRTWStateStorageClass=Auto  FilterContinuousStateAttributes=''  FilterStateMustResolveToSignalObject=off  FilterRTWStateStorageClass=Auto  ParallelPVariant=InternalParameters  IdealPVariant=Disabled  IVariant=InternalParameters  DVariant=InternalParameters  IntegratorVariant=Continuous  SatVariant=Disabled  AWVariant=Passthrough  PCopyVariant=Disabled  TRVariant=Disabled  FdbkBlocksVariant=Forward  IdealPFdbkVariant=Disabled  SatFdbkVariant=Disabled  DerivativeFilterVariant=ContFilter  NVariant=InternalParameters  NCopyVariant=Disabled  FilterICVariant=InternalICsFilter  IntegratorICVariant=InternalICs  ExternalResetVariant=Disabled  TRSumVariant=Passthrough  SumFdbkVariant=Disabled  SumVariant=Sum_PID  TsampFilterVariant=InternalTs  TsampNgainVariant=Passthrough  TsampIntegralVariant=Disabled_SignalSpec  ExternalSaturationOutDataTypeStr=Inherit: Same as second input
  Sign1 : Signum
  Sign2 : Signum
  Sum : Sum  Inputs=++|
  Sum{1,3,6,8} (4 alike) : Sum  Inputs=|++
  Sum2 : Sum  Inputs=|+-
  Sum4 : Sum  Inputs=|+-
  Sum5 : Sum  Inputs=|+-
  Switch : Switch  Criteria=u2 > Threshold  SaturateOnIntegerOverflow=off  InputSameDT=off
  diff: delta_e : Outport
  diff:  delta_a : Outport  Port=2
  diff: delta_r : Outport  Port=3
  diff:  Tcom : Outport  Port=4
  wires:
  Bus Selector3/1 -> Gain6/1, Sum5/2  "<p>"
  Sum4/1 -> Gain5/1
  Bus Selector3/2 -> Gain2/1, Sum2/2  "<q>"
  Bus Selector3/3 -> Sum4/2, Gain4/1  "<r>"
  q_cmd/1 -> Sum2/1
  "p, q, r, phi, theta"/1 -> Bus Selector3/1
  p_cmd/1 -> Sum5/1, Abs1/1
  r_cmd/1 -> Sum4/1, Abs2/1
  Sum1/1 -> diff: delta_e/1
  Tcom+/1 -> diff:  Tcom/1
  Sum2/1 -> Gain1/1, Gain/1
  Gain/1 -> Sum/2
  Sum/1 -> Sum1/1
  Gain1/1 -> Integrator/1
  Integrator/1 -> Sum/1
  Gain2/1 -> Sum1/2
  Sum3/1 -> diff:  delta_a/1
  Gain4/1 -> Sum3/2
  Gain5/1 -> Sum8/1
  Sum6/1 -> diff: delta_r/1
  Gain6/1 -> Sum6/2
  Sum5/1 -> Gain3/1
  Bus Selector3/4 -> PID Controller/1  "<phi>"
  Gain3/1 -> Sum3/1
  Sum8/1 -> Sum6/1
  PID Controller/1 -> Switch/3
  Sign1/1 -> OR/2
  Sign2/1 -> OR/1
  GreaterThan2/1 -> Sign1/1
  Constant/1 -> GreaterThan2/2
  Abs2/1 -> GreaterThan2/1
  Constant1/1 -> GreaterThan1/2
  Abs1/1 -> GreaterThan1/1
  GreaterThan1/1 -> Sign2/1
  Constant2/1 -> Switch/1
  Switch/1 -> Sum8/2
  OR/1 -> Switch/2

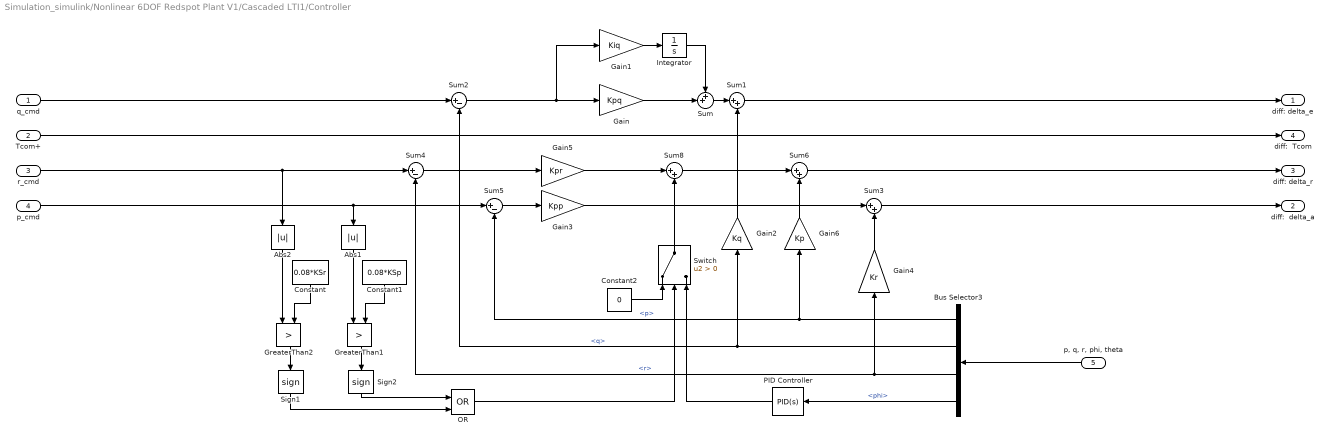
== system Simulation_simulink/Nonlinear 6DOF Redspot Plant V1/Cascaded LTI1/Controller ==
  q_cmd : Inport
  Tcom+ : Inport  Port=2
  r_cmd : Inport  Port=3
  p_cmd : Inport  Port=4
  "p, q, r, phi, theta" : Inport  Port=5
  Abs1 : Abs  SaturateOnIntegerOverflow=off
  Abs2 : Abs  SaturateOnIntegerOverflow=off
  Bus Selector3 : BusSelector  OutputSignals=p,q,r,phi
  Constant : Constant  Value=0.08*KSr
  Constant1 : Constant  Value=0.08*KSp
  Constant2 : Constant  Value=0
  Gain : Gain  Gain=Kpq
  Gain1 : Gain  Gain=Kiq
  Gain2 : Gain  Gain=Kq
  Gain3 : Gain  Gain=Kpp
  Gain4 : Gain  Gain=Kr
  Gain5 : Gain  Gain=Kpr
  Gain6 : Gain  Gain=Kp
  GreaterThan1 : RelationalOperator  Operator=>  OutDataTypeStr=boolean  RndMeth=Simplest  InputSameDT=off
  GreaterThan2 : RelationalOperator  Operator=>  OutDataTypeStr=boolean  RndMeth=Simplest  InputSameDT=off
  Integrator : Integrator
  OR : Logic  Operator=OR  IconShape=distinctive  AllPortsSameDT=off  OutDataTypeStr=boolean
  PID Controller : slpidlib/PID Controller  Controller=PID  Form=Parallel  TimeDomain=Continuous-time  UseExternalTs=off  SampleTime=-1  IntegratorMethod=Forward Euler  FilterMethod=Forward Euler  ControllerParametersSource=internal  P=10  I=0.5  UseKiTs=off  D=5  N=100  UseFilter=on  TunerSelectOption=Transfer Function Based (PID Tuner App)  InitialConditionSource=internal  InitialConditionForIntegrator=0  InitialConditionForFilter=0  DifferentiatorICPrevScaledInput=0  ExternalReset=none  TrackingMode=off  Kt=1  LimitOutput=off  SatLimitsSource=internal  UpperSaturationLimit=inf  LowerSaturationLimit=-inf  LinearizeAsGain=on  AntiWindupMode=none  Kb=1  LimitIntegrator=off  UpperIntegratorSaturationLimit=inf  LowerIntegratorSaturationLimit=-inf  POutMin=[]  POutMax=[]  IOutMin=[]  IOutMax=[]  DOutMin=[]  DOutMax=[]  NOutMin=[]  NOutMax=[]  SumOutMin=[]  SumOutMax=[]  SaturationOutMin=[]  SaturationOutMax=[]  PParamMin=[]  PParamMax=[]  IParamMin=[]  IParamMax=[]  DParamMin=[]  DParamMax=[]  NParamMin=[]  NParamMax=[]  KbParamMin=[]  KbParamMax=[]  KtParamMin=[]  KtParamMax=[]  KbOutMin=[]  KbOutMax=[]  KtOutMin=[]  KtOutMax=[]  IntegratorOutMin=[]  IntegratorOutMax=[]  FilterOutMin=[]  FilterOutMax=[]  SumI1OutMin=[]  SumI1OutMax=[]  SumI2OutMin=[]  SumI2OutMax=[]  SumI3OutMin=[]  SumI3OutMax=[]  SumI4OutMin=[]  SumI4OutMax=[]  SumDOutMin=[]  SumDOutMax=[]  DifferentiatorOutMin=[]  DifferentiatorOutMax=[]  FilterDiffOutCoefMin=[]  FilterDiffOutCoefMax=[]  ReciprocalOutMin=[]  ReciprocalOutMax=[]  SumDenOutMin=[]  SumDenOutMax=[]  SumNumOutMin=[]  SumNumOutMax=[]  DivideOutMin=[]  DivideOutMax=[]  UdiffTsProdOutMin=[]  UdiffTsProdOutMax=[]  NTsProdOutMin=[]  NTsProdOutMax=[]  UintegralTsProdOutMin=[]  UintegralTsProdOutMax=[]  UngainTsProdOutMin=[]  UngainTsProdOutMax=[]  ClampingZeroOutDataTypeStr=Inherit: Inherit via back propagation  ClampingZeroOutMin=[]  ClampingZeroOutMax=[]  FilterDenConstantOutDataTypeStr=Inherit: Inherit via back propagation  FilterDenConstantOutMin=[]  FilterDenConstantOutMax=[]  PCopyOutDataTypeStr=Inherit: Inherit via back propagation  PCopyOutMin=[]  PCopyOutMax=[]  NCopyOutDataTypeStr=Inherit: Inherit via back propagation  NCopyOutMin=[]  NCopyOutMax=[]  IntegratorContinuousStateAttributes=''  IntegratorStateMustResolveToSignalObject=off  IntegratorRTWStateStorageClass=Auto  FilterContinuousStateAttributes=''  FilterStateMustResolveToSignalObject=off  FilterRTWStateStorageClass=Auto  ParallelPVariant=InternalParameters  IdealPVariant=Disabled  IVariant=InternalParameters  DVariant=InternalParameters  IntegratorVariant=Continuous  SatVariant=Disabled  AWVariant=Passthrough  PCopyVariant=Disabled  TRVariant=Disabled  FdbkBlocksVariant=Forward  IdealPFdbkVariant=Disabled  SatFdbkVariant=Disabled  DerivativeFilterVariant=ContFilter  NVariant=InternalParameters  NCopyVariant=Disabled  FilterICVariant=InternalICsFilter  IntegratorICVariant=InternalICs  ExternalResetVariant=Disabled  TRSumVariant=Passthrough  SumFdbkVariant=Disabled  SumVariant=Sum_PID  TsampFilterVariant=InternalTs  TsampNgainVariant=Passthrough  TsampIntegralVariant=Disabled_SignalSpec  ExternalSaturationOutDataTypeStr=Inherit: Same as second input
  Sign1 : Signum
  Sign2 : Signum
  Sum : Sum  Inputs=++|
  Sum{1,3,6,8} (4 alike) : Sum  Inputs=|++
  Sum2 : Sum  Inputs=|+-
  Sum4 : Sum  Inputs=|+-
  Sum5 : Sum  Inputs=|+-
  Switch : Switch  Criteria=u2 > Threshold  SaturateOnIntegerOverflow=off  InputSameDT=off
  diff: delta_e : Outport
  diff:  delta_a : Outport  Port=2
  diff: delta_r : Outport  Port=3
  diff:  Tcom : Outport  Port=4
  wires:
  Bus Selector3/1 -> Gain6/1, Sum5/2  "<p>"
  Sum4/1 -> Gain5/1
  Bus Selector3/2 -> Gain2/1, Sum2/2  "<q>"
  Bus Selector3/3 -> Sum4/2, Gain4/1  "<r>"
  q_cmd/1 -> Sum2/1
  "p, q, r, phi, theta"/1 -> Bus Selector3/1
  p_cmd/1 -> Sum5/1, Abs1/1
  r_cmd/1 -> Sum4/1, Abs2/1
  Sum1/1 -> diff: delta_e/1
  Tcom+/1 -> diff:  Tcom/1
  Sum2/1 -> Gain1/1, Gain/1
  Gain/1 -> Sum/2
  Sum/1 -> Sum1/1
  Gain1/1 -> Integrator/1
  Integrator/1 -> Sum/1
  Gain2/1 -> Sum1/2
  Sum3/1 -> diff:  delta_a/1
  Gain4/1 -> Sum3/2
  Gain5/1 -> Sum8/1
  Sum6/1 -> diff: delta_r/1
  Gain6/1 -> Sum6/2
  Sum5/1 -> Gain3/1
  Bus Selector3/4 -> PID Controller/1  "<phi>"
  Gain3/1 -> Sum3/1
  Sum8/1 -> Sum6/1
  PID Controller/1 -> Switch/3
  Sign1/1 -> OR/2
  Sign2/1 -> OR/1
  GreaterThan2/1 -> Sign1/1
  Constant/1 -> GreaterThan2/2
  Abs2/1 -> GreaterThan2/1
  Constant1/1 -> GreaterThan1/2
  Abs1/1 -> GreaterThan1/1
  GreaterThan1/1 -> Sign2/1
  Constant2/1 -> Switch/1
  Switch/1 -> Sum8/2
  OR/1 -> Switch/2

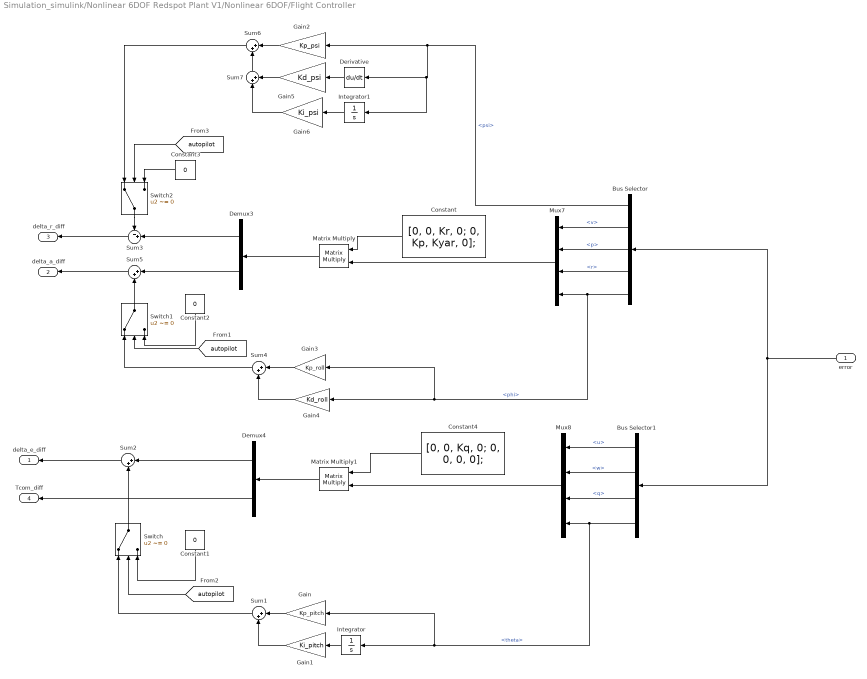
== system Simulation_simulink/Nonlinear 6DOF Redspot Plant V1/Nonlinear 6DOF/Flight Controller ==
  error : Inport
  Bus Selector : BusSelector  OutputSignals=psi,v,p,r,phi
  Bus Selector1 : BusSelector  OutputSignals=u,w,q,theta
  Constant : Constant  Value=|
      | [0,  0, Kr, 0;
      | 0, Kp, Kyar, 0];
  Constant1 : Constant  Value=0
  Constant2 : Constant  Value=0
  Constant3 : Constant  Value=0
  Constant4 : Constant  Value="[0, 0, Kq, 0; 0, 0,  0, 0];"
  Demux3 : Demux  Outputs=2
  Demux4 : Demux  Outputs=2
  Derivative : Derivative
  Gain : Gain  Gain=Kp_pitch
  Gain1 : Gain  Gain=Ki_pitch
  Gain2 : Gain  Gain=Kp_psi
  Gain3 : Gain  Gain=Kp_roll
  Gain4 : Gain  Gain=Kd_roll
  Gain5 : Gain  Gain=Kd_psi
  Gain6 : Gain  Gain=Ki_psi
  Integrator : Integrator
  Integrator1 : Integrator  ContinuousStateAttributes='psi_error'
  Matrix Multiply : Product  Multiplication=Matrix(*)
  Matrix Multiply1 : Product  Multiplication=Matrix(*)
  Mux7 : Mux
  Mux8 : Mux
  Sum{1..2,4..7} (6 alike) : Sum  Inputs=|++
  Sum3 : Sum  Inputs=-+|
  Switch : Switch  Criteria=u2 ~= 0  SaturateOnIntegerOverflow=off  InputSameDT=off
  Switch1 : Switch  Criteria=u2 ~= 0  SaturateOnIntegerOverflow=off  InputSameDT=off
  Switch2 : Switch  Criteria=u2 ~= 0  SaturateOnIntegerOverflow=off  InputSameDT=off
  delta_e_diff : Outport
  delta_a_diff : Outport  Port=2
  delta_r_diff : Outport  Port=3
  Tcom_diff : Outport  Port=4
  wires:
  Bus Selector1/3 -> Mux8/3  "<q>"
  Matrix Multiply1/1 -> Demux4/1
  Demux3/2 -> Sum5/1
  Bus Selector/3 -> Mux7/2  "<p>"
  Mux8/1 -> Matrix Multiply1/2
  Bus Selector/4 -> Mux7/3  "<r>"
  Sum2/1 -> delta_e_diff/1
  error/1 -> Bus Selector/1, Bus Selector1/1
  Demux4/2 -> Tcom_diff/1
  Mux7/1 -> Matrix Multiply/2
  Bus Selector/2 -> Mux7/1  "<v>"
  Bus Selector1/2 -> Mux8/2  "<w>"
  Bus Selector1/1 -> Mux8/1  "<u>"
  Bus Selector1/4 -> Integrator/1, Gain/1, Mux8/4  "<theta>"
  Matrix Multiply/1 -> Demux3/1
  Gain/1 -> Sum1/1
  Integrator/1 -> Gain1/1
  Gain1/1 -> Sum1/2
  Sum1/1 -> Switch/1
  Demux4/1 -> Sum2/1
  Bus Selector/5 -> Mux7/4, Gain4/1, Gain3/1  "<phi>"
  Gain4/1 -> Sum4/2
  Gain3/1 -> Sum4/1
  Sum5/1 -> delta_a_diff/1
  Switch/1 -> Sum2/2
  [autopilot] -> Switch/2
  Constant1/1 -> Switch/3
  Constant2/1 -> Switch1/3
  [autopilot] -> Switch1/2
  Sum4/1 -> Switch1/1
  Switch1/1 -> Sum5/2
  Demux3/1 -> Sum3/2
  Sum3/1 -> delta_r_diff/1
  Sum6/1 -> Switch2/1
  Switch2/1 -> Sum3/1
  [autopilot] -> Switch2/2
  Constant3/1 -> Switch2/3
  Bus Selector/1 -> Derivative/1, Integrator1/1, Gain2/1  "<psi>"
  Gain2/1 -> Sum6/1
  Integrator1/1 -> Gain6/1
  Gain6/1 -> Sum7/1
  Gain5/1 -> Sum7/2
  Sum7/1 -> Sum6/2
  Derivative/1 -> Gain5/1
  Constant4/1 -> Matrix Multiply1/1
  Constant/1 -> Matrix Multiply/1

== matlab function Simulation_simulink/Nonlinear 6DOF Redspot Plant V1/Augmented LTI (lateral + longitudinal)/MATLAB Function ==
  data: Vb input; Xe_dot output; euler input
function Xe_dot = integrate_Xe(Vb, euler)

u = Vb(1);
v = Vb(2);
w = Vb(3);

e1 = euler(1);
e2 = euler(2);
e3 = euler(3);

Xe_dot = [cos(e2)*cos(e3)*u + (sin(e1)*sin(e2)*cos(e3) - cos(e1)*sin(e3))*v + (cos(e1)*sin(e2)*cos(e3) + sin(e1)*sin(e3))*w; ...
          cos(e2)*sin(e3)*u + (sin(e1)*sin(e2)*sin(e3) + cos(e1)*cos(e3))*v + (cos(e1)*sin(e2)*sin(e3) - sin(e1)*cos(e3))*w; ...
               (-sin(e2))*u +                             sin(e1)*cos(e2)*v +                             cos(e1)*cos(e2)*w];


end
